simulink model "sffwm"  (R2024b)
settings: Solver=VariableStepAuto  StartTime=0.0  StopTime=inf  RelTol=1e-3
settings Model: Creator=Thanu  LastModifiedBy=HP

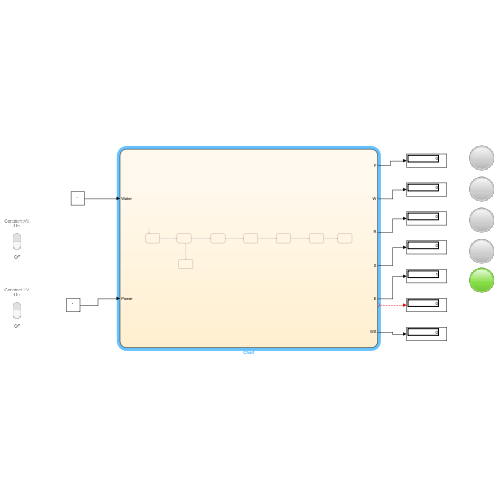
[thumbnail: Simulink's stored preview of the top-level diagram]
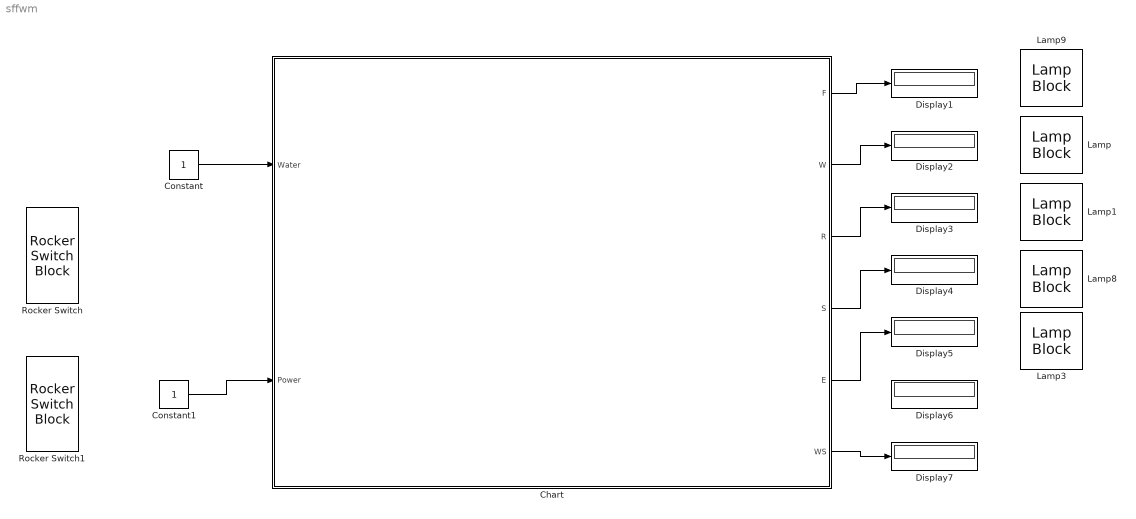
== system sffwm ==
  Chart : Stateflow chart  TreatAsAtomicUnit=on
  Constant : Constant
  Constant1 : Constant
  Display{1..7} (7 alike) : Display
  Lamp{,1,3,8..9} (5 alike) : LampBlock  LabelPosition=Hide
  Rocker Switch : RockerSwitchBlock
      settings: Values={{'Off', 'On'}, [0 1]}
  Rocker Switch1 : RockerSwitchBlock
      settings: Values={{'Off', 'On'}, [0 1]}
  wires:
  Chart/6(WS) -> Display7/1
  ? -> Display6/1
  Chart/1(F) -> Display1/1
  Chart/3(R) -> Display3/1
  Chart/2(W) -> Display2/1
  Chart/4(S) -> Display4/1
  Chart/5(E) -> Display5/1
  Constant/1 -> Chart/1(Water)
  Constant1/1 -> Chart/2(Power)

== stateflow chart sffwm/Chart ==
  state Idle
  state Water_Supply
  state Fill
    entry:F=1;
  state Washing
    entry:F=0,W=1;
  state Rinse
    entry:W=0,R=1;
  state Spin
    entry:R=0,S=1;
  state End
    entry:S=0,E=1
  state Water_Indicator
    entry:WS=1;
  (default) -> Idle
  Idle -> Water_Supply : [Power==1]
  Water_Supply -> Fill [order 1] : [Water==1]
  Fill -> Washing : after(10,sec)
  Washing -> Rinse : after(10,sec)
  Rinse -> Spin : after(10,sec)
  Spin -> End : after(5,sec)
  Water_Supply -> Water_Indicator [order 2] : [Water==0]
  data: Water input; Power input; F output; W output; R output; S output; E output; WS output
